simulink model "CM620C_MotAg0Meas"  (R2013b)
settings: Solver=FixedStepDiscrete  SolverMode=SingleTasking  StartTime=0.0  StopTime=1  FixedStep=0.0000625  RelTol=1e-3
values from neighbouring files (symbols this model uses):
  ARCHGLBPRM_2PI_ULS_F32 = DataDict.Constant    [CM620C_MotAg0Meas_DataDict.m]
  COEFFTBLELMSIZE_CNT_U08 = DataDict.Constant    [CM620C_MotAg0Meas_DataDict.m]
  COEFFTBLSIZE_CNT_U08 = DataDict.Constant    [CM620C_MotAg0Meas_DataDict.m]
  CORRNTBLAGSTEPSIZE_MATRAD_F32 = DataDict.Constant    [CM620C_MotAg0Meas_DataDict.m]
  CORRNTBLSIDXOFFS_CNT_U16 = DataDict.Constant    [CM620C_MotAg0Meas_DataDict.m]
  CORRNTBLSIZE_CNT_U16 = DataDict.Constant    [CM620C_MotAg0Meas_DataDict.m]
  CORRNTBLSIZEMASK_CNT_U08 = DataDict.Constant    [CM620C_MotAg0Meas_DataDict.m]
  MOTAG0ERRTHD_MOTREV_U0P16 = DataDict.Constant    [CM620C_MotAg0Meas_DataDict.m]
  MotAg0PrtclFlt = DataDict.NTC    [CM620C_MotAg0Meas_DataDict.m]
  MOTAG0PRTCLFLTFAILSTEP_CNT_U16 = DataDict.Constant    [CM620C_MotAg0Meas_DataDict.m]
  MOTAG0PRTCLFLTPASSSTEP_CNT_U16 = DataDict.Constant    [CM620C_MotAg0Meas_DataDict.m]
  MOTAGCPTLIMFLTMASK_CNT_U32 = DataDict.Constant    [CM620C_MotAg0Meas_DataDict.m]
  MOTAGDELTAPERCORRNPT_CNT_U16 = DataDict.Constant    [CM620C_MotAg0Meas_DataDict.m]
  MOTAGFLTMASK_CNT_U32 = DataDict.Constant    [CM620C_MotAg0Meas_DataDict.m]
  MOTAGIDXMASK_CNT_U16 = DataDict.Constant    [CM620C_MotAg0Meas_DataDict.m]
  MOTAGLIMMASK_CNT_S32 = DataDict.Constant    [CM620C_MotAg0Meas_DataDict.m]
  MOTAGMGNLIMFLTMASK_CNT_U32 = DataDict.Constant    [CM620C_MotAg0Meas_DataDict.m]
  MOTAGMINWAITPERD_CNT_U32 = DataDict.Constant    [CM620C_MotAg0Meas_DataDict.m]
  MOTAGOFFS_CNT_S32 = DataDict.Constant    [CM620C_MotAg0Meas_DataDict.m]
  MOTAGOVFFLTMASK_CNT_U32 = DataDict.Constant    [CM620C_MotAg0Meas_DataDict.m]
  MOTAGSPITRSMMASK_CNT_U32 = DataDict.Constant    [CM620C_MotAg0Meas_DataDict.m]
  MOTAGVLTGFLTMASK_CNT_U32 = DataDict.Constant    [CM620C_MotAg0Meas_DataDict.m]
  NOMOTAGFLTMASK_CNT_U32 = DataDict.Constant    [CM620C_MotAg0Meas_DataDict.m]
  READBUFADR_CNT_U32 = DataDict.Constant    [CM620C_MotAg0Meas_DataDict.m]
  READBUFIDX_CNT_U08 = DataDict.Constant    [CM620C_MotAg0Meas_DataDict.m]
  SNSRAGMASK_CNT_U32 = DataDict.Constant    [CM620C_MotAg0Meas_DataDict.m]
  SNSRCNTMASK_CNT_U32 = DataDict.Constant    [CM620C_MotAg0Meas_DataDict.m]
  SPIAGCNTREGIDX_CNT_U08 = DataDict.Constant    [CM620C_MotAg0Meas_DataDict.m]
  SPIAGREGIDX_CNT_U08 = DataDict.Constant    [CM620C_MotAg0Meas_DataDict.m]
  SPISTATREGIDX_CNT_U08 = DataDict.Constant    [CM620C_MotAg0Meas_DataDict.m]
  SPITURNCNTRREGIDX_CNT_U08 = DataDict.Constant    [CM620C_MotAg0Meas_DataDict.m]
  STRTPTRINITVAL_CNT_U32 = DataDict.Constant    [CM620C_MotAg0Meas_DataDict.m]
  STRTPTRPERVAL_CNT_U32 = DataDict.Constant    [CM620C_MotAg0Meas_DataDict.m]
  TURNCNTRHALFOFFS_CNT_S16 = DataDict.Constant    [CM620C_MotAg0Meas_DataDict.m]
  TURNCNTROFFS_CNT_S16 = DataDict.Constant    [CM620C_MotAg0Meas_DataDict.m]
  TURNCNTRREGMASK_CNT_U32 = DataDict.Constant    [CM620C_MotAg0Meas_DataDict.m]
  VLDMOTAGFLTMASK_CNT_U32 = DataDict.Constant    [CM620C_MotAg0Meas_DataDict.m]
undefined symbols (not defined in the file or in its folder): NtcSts1, sigbuilder_block
libraries: simulink x41, FloatToFixd x1, NxtrMax x1
(part 5 of 7)

== system CM620C_MotAg0Meas/MotAg0Meas/MotAg0MeasPer2/MotAg0Calcn/MotAg0Processing/Diagnostics/SetParamByte/Boolean to u8   ==
  InputBoolean : Inport  OutDataTypeStr=boolean
  CopyRight2 : Subsystem  Description=|  mask(Copyright Information){none=on}
      | Copyright info block.                                               
      |                                                                     
      | Place copyright information at the top of every subsystem in design.
      mask prompts: none "No parameters"
      mask help: Place copyright information at the top of every subsystem in design.
      mask Display:
      | NxtrConf = 'Nexteer Confidential';
      | 
      | sys = bdroot; %handle for the current model ("system")
      | first = get_param(sys,'Created');
      | first = first(end-3:end);  %year is last four digits
      | 
      | last = get_param(sys,'LastModifiedDate');
      | if isempty(last)
      |     last = datestr(now,'yyyy');
      | else
      |     last = last(end-3:end);
      | end
      | 
      | if strcmp(first,last)
      |     fprintf('%s -- Copyright %s Nexteer',NxtrConf,first)
      | else
      |     fprintf('%s -- %s%s- %s Nexteer',NxtrConf,char(169),first,last)
      | end
  If : If  IfExpression=u1 ~= 0
  Merge : Merge
  Output 0 : Subsystem  TreatAsAtomicUnit=on
  Output 1 : Subsystem  TreatAsAtomicUnit=on
  OutputNumber : Outport  OutDataTypeStr=uint8
  wires:
  InputBoolean/1 -> If/1
  If/1 -> Output 1/Action
  If/2 -> Output 0/Action
  Output 1/1(Out1) -> Merge/1
  Output 0/1(Out1) -> Merge/2
  Merge/1 -> OutputNumber/1

== system CM620C_MotAg0Meas/MotAg0Meas/MotAg0MeasPer2/MotAg0Calcn/MotAg0Processing/Diagnostics/SetParamByte/Boolean to u8    ==
  InputBoolean : Inport  OutDataTypeStr=boolean
  CopyRight2 : Subsystem  Description=|  mask(Copyright Information){none=on}
      | Copyright info block.                                               
      |                                                                     
      | Place copyright information at the top of every subsystem in design.
      mask prompts: none "No parameters"
      mask help: Place copyright information at the top of every subsystem in design.
      mask Display:
      | NxtrConf = 'Nexteer Confidential';
      | 
      | sys = bdroot; %handle for the current model ("system")
      | first = get_param(sys,'Created');
      | first = first(end-3:end);  %year is last four digits
      | 
      | last = get_param(sys,'LastModifiedDate');
      | if isempty(last)
      |     last = datestr(now,'yyyy');
      | else
      |     last = last(end-3:end);
      | end
      | 
      | if strcmp(first,last)
      |     fprintf('%s -- Copyright %s Nexteer',NxtrConf,first)
      | else
      |     fprintf('%s -- %s%s- %s Nexteer',NxtrConf,char(169),first,last)
      | end
  If : If  IfExpression=u1 ~= 0
  Merge : Merge
  Output 0 : Subsystem  TreatAsAtomicUnit=on
  Output 1 : Subsystem  TreatAsAtomicUnit=on
  OutputNumber : Outport  OutDataTypeStr=uint8
  wires:
  Merge/1 -> OutputNumber/1
  Output 0/1(Out1) -> Merge/2
  Output 1/1(Out1) -> Merge/1
  If/2 -> Output 0/Action
  If/1 -> Output 1/Action
  InputBoolean/1 -> If/1

== system CM620C_MotAg0Meas/MotAg0Meas/MotAg0MeasPer2/MotAg0Calcn/MotAg0Processing/Diagnostics/SetParamByte/Boolean to u8     ==
  InputBoolean : Inport  OutDataTypeStr=boolean
  CopyRight2 : Subsystem  Description=|  mask(Copyright Information){none=on}
      | Copyright info block.                                               
      |                                                                     
      | Place copyright information at the top of every subsystem in design.
      mask prompts: none "No parameters"
      mask help: Place copyright information at the top of every subsystem in design.
      mask Display:
      | NxtrConf = 'Nexteer Confidential';
      | 
      | sys = bdroot; %handle for the current model ("system")
      | first = get_param(sys,'Created');
      | first = first(end-3:end);  %year is last four digits
      | 
      | last = get_param(sys,'LastModifiedDate');
      | if isempty(last)
      |     last = datestr(now,'yyyy');
      | else
      |     last = last(end-3:end);
      | end
      | 
      | if strcmp(first,last)
      |     fprintf('%s -- Copyright %s Nexteer',NxtrConf,first)
      | else
      |     fprintf('%s -- %s%s- %s Nexteer',NxtrConf,char(169),first,last)
      | end
  If : If  IfExpression=u1 ~= 0
  Merge : Merge
  Output 0 : Subsystem  TreatAsAtomicUnit=on
  Output 1 : Subsystem  TreatAsAtomicUnit=on
  OutputNumber : Outport  OutDataTypeStr=uint8
  wires:
  InputBoolean/1 -> If/1
  If/1 -> Output 1/Action
  If/2 -> Output 0/Action
  Output 1/1(Out1) -> Merge/1
  Output 0/1(Out1) -> Merge/2
  Merge/1 -> OutputNumber/1

== system CM620C_MotAg0Meas/MotAg0Meas/MotAg0MeasPer2/MotAg0Calcn/MotAg0Processing/Diagnostics/SetParamByte/Boolean to u8      ==
  InputBoolean : Inport  OutDataTypeStr=boolean
  CopyRight2 : Subsystem  Description=|  mask(Copyright Information){none=on}
      | Copyright info block.                                               
      |                                                                     
      | Place copyright information at the top of every subsystem in design.
      mask prompts: none "No parameters"
      mask help: Place copyright information at the top of every subsystem in design.
      mask Display:
      | NxtrConf = 'Nexteer Confidential';
      | 
      | sys = bdroot; %handle for the current model ("system")
      | first = get_param(sys,'Created');
      | first = first(end-3:end);  %year is last four digits
      | 
      | last = get_param(sys,'LastModifiedDate');
      | if isempty(last)
      |     last = datestr(now,'yyyy');
      | else
      |     last = last(end-3:end);
      | end
      | 
      | if strcmp(first,last)
      |     fprintf('%s -- Copyright %s Nexteer',NxtrConf,first)
      | else
      |     fprintf('%s -- %s%s- %s Nexteer',NxtrConf,char(169),first,last)
      | end
  If : If  IfExpression=u1 ~= 0
  Merge : Merge
  Output 0 : Subsystem  TreatAsAtomicUnit=on
  Output 1 : Subsystem  TreatAsAtomicUnit=on
  OutputNumber : Outport  OutDataTypeStr=uint8
  wires:
  Merge/1 -> OutputNumber/1
  Output 0/1(Out1) -> Merge/2
  Output 1/1(Out1) -> Merge/1
  If/2 -> Output 0/Action
  If/1 -> Output 1/Action
  InputBoolean/1 -> If/1

== system CM620C_MotAg0Meas/MotAg0Meas/MotAg0MeasPer2/MotAg0Calcn/MotAg0Processing/Diagnostics/SetParamByte/Boolean to uint8 ==
  InputBoolean : Inport  OutDataTypeStr=boolean
  CopyRight2 : Subsystem  Description=|  mask(Copyright Information){none=on}
      | Copyright info block.                                               
      |                                                                     
      | Place copyright information at the top of every subsystem in design.
      mask prompts: none "No parameters"
      mask help: Place copyright information at the top of every subsystem in design.
      mask Display:
      | NxtrConf = 'Nexteer Confidential';
      | 
      | sys = bdroot; %handle for the current model ("system")
      | first = get_param(sys,'Created');
      | first = first(end-3:end);  %year is last four digits
      | 
      | last = get_param(sys,'LastModifiedDate');
      | if isempty(last)
      |     last = datestr(now,'yyyy');
      | else
      |     last = last(end-3:end);
      | end
      | 
      | if strcmp(first,last)
      |     fprintf('%s -- Copyright %s Nexteer',NxtrConf,first)
      | else
      |     fprintf('%s -- %s%s- %s Nexteer',NxtrConf,char(169),first,last)
      | end
  If : If  IfExpression=u1 ~= 0
  Merge : Merge
  Output 0 : Subsystem  TreatAsAtomicUnit=on
  Output 1 : Subsystem  TreatAsAtomicUnit=on
  OutputNumber : Outport  OutDataTypeStr=uint8
  wires:
  Merge/1 -> OutputNumber/1
  Output 0/1(Out1) -> Merge/2
  Output 1/1(Out1) -> Merge/1
  If/2 -> Output 0/Action
  If/1 -> Output 1/Action
  InputBoolean/1 -> If/1

== system CM620C_MotAg0Meas/MotAg0Meas/MotAg0MeasPer2/MotAg0Calcn/MotAg0Processing/Diagnostics/SetParamByte/CopyRight2 ==

== system CM620C_MotAg0Meas/MotAg0Meas/MotAg0MeasPer2/MotAg0Calcn/MotAg0Processing/Diagnostics/SetParamByte/Subsystem1 ==
  Test_Lgc : Inport
  MotAg0SyncErr : Inport  Port=2
  MotAg0NoAg : Inport  Port=3
  MotAg0NoXY : Inport  Port=4
  MotAg0OutofLim : Inport  Port=5
  MotAg0XYOutofLim : Inport  Port=6
  MotAg0DSPOverFlow : Inport  Port=7
  MotAg0VltgFlt : Inport  Port=8
  CopyRight2 : Subsystem  Description=|  mask(Copyright Information){none=on}
      | Copyright info block.                                               
      |                                                                     
      | Place copyright information at the top of every subsystem in design.
      mask prompts: none "No parameters"
      mask help: Place copyright information at the top of every subsystem in design.
      mask Display:
      | NxtrConf = 'Nexteer Confidential';
      | 
      | sys = bdroot; %handle for the current model ("system")
      | first = get_param(sys,'Created');
      | first = first(end-3:end);  %year is last four digits
      | 
      | last = get_param(sys,'LastModifiedDate');
      | if isempty(last)
      |     last = datestr(now,'yyyy');
      | else
      |     last = last(end-3:end);
      | end
      | 
      | if strcmp(first,last)
      |     fprintf('%s -- Copyright %s Nexteer',NxtrConf,first)
      | else
      |     fprintf('%s -- %s%s- %s Nexteer',NxtrConf,char(169),first,last)
      | end
  If : If  IfExpression=u1==1
  Merge : Merge
  No Fault : Subsystem  TreatAsAtomicUnit=on
  Scope : Scope
      settings: SaveName=ScopeData11
  Set ParamByte : Subsystem  TreatAsAtomicUnit=on
  ParamByte : Outport
  wires:
  MotAg0NoAg/1 -> Set ParamByte/1(MotAg0NoAg)
  MotAg0NoXY/1 -> Set ParamByte/2(MotAg0NoXY)
  MotAg0OutofLim/1 -> Set ParamByte/3(MotAg0OutofLim)
  MotAg0XYOutofLim/1 -> Set ParamByte/4(MotAg0XYOutofLim)
  MotAg0DSPOverFlow/1 -> Set ParamByte/5(MotAg0DSPOverFlow)
  MotAg0VltgFlt/1 -> Set ParamByte/6(MotAg0VltgFlt)
  Test_Lgc/1 -> If/1
  MotAg0SyncErr/1 -> Set ParamByte/7(MotAg0SyncErr)
  If/1 -> Set ParamByte/Action
  If/2 -> No Fault/Action
  Set ParamByte/1(ParamByte) -> Merge/1
  No Fault/1(ParamByte) -> Merge/2
  Merge/1 -> Scope/1, ParamByte/1

== system CM620C_MotAg0Meas/MotAg0Meas/MotAg0MeasPer2/MotAg0Calcn/MotAg0Processing/Offset Compensation /First Time Offset Calcn/CopyRight2 ==

== system CM620C_MotAg0Meas/MotAg0Meas/MotAg0MeasPer2/MotAg0Calcn/MotAg0Processing/Offset Compensation /Rt Offs Calcn/CopyRight2 ==

== system CM620C_MotAg0Meas/MotAg0Meas/MotAg0MeasPer2/MotAg0Calcn/MotAg0Processing/SPI  Motor Angle Calcn/Polarity Correction/CopyRight1 ==

== system CM620C_MotAg0Meas/MotAg0Meas/MotAg0MeasPer2/MotAg0Calcn/MotAg0Processing/SPI  Motor Angle Calcn/Polarity Correction/Negative Polarity ==
  MotAg0RawSpiMecl : Inport
  Action Port : ActionPort  ActionType=then
  Constant : Constant  Value=65535  OutDataTypeStr=uint16
  CopyRight2 : Subsystem  Description=|  mask(Copyright Information){none=on}
      | Copyright info block.                                               
      |                                                                     
      | Place copyright information at the top of every subsystem in design.
      mask prompts: none "No parameters"
      mask help: Place copyright information at the top of every subsystem in design.
      mask Display:
      | NxtrConf = 'Nexteer Confidential';
      | 
      | sys = bdroot; %handle for the current model ("system")
      | first = get_param(sys,'Created');
      | first = first(end-3:end);  %year is last four digits
      | 
      | last = get_param(sys,'LastModifiedDate');
      | if isempty(last)
      |     last = datestr(now,'yyyy');
      | else
      |     last = last(end-3:end);
      | end
      | 
      | if strcmp(first,last)
      |     fprintf('%s -- Copyright %s Nexteer',NxtrConf,first)
      | else
      |     fprintf('%s -- %s%s- %s Nexteer',NxtrConf,char(169),first,last)
      | end
  Subtract : Sum  Inputs=+-
  MotAg0SpiPolarityCorrd : Outport
  wires:
  Constant/1 -> Subtract/1
  MotAg0RawSpiMecl/1 -> Subtract/2
  Subtract/1 -> MotAg0SpiPolarityCorrd/1

== system CM620C_MotAg0Meas/MotAg0Meas/MotAg0MeasPer2/MotAg0Calcn/MotAg0Processing/SPI  Motor Angle Calcn/Polarity Correction/Positive Polarity ==
  MotAg0RawSpiMecl : Inport
  Action Port : ActionPort  ActionType=else
  CopyRight2 : Subsystem  Description=|  mask(Copyright Information){none=on}
      | Copyright info block.                                               
      |                                                                     
      | Place copyright information at the top of every subsystem in design.
      mask prompts: none "No parameters"
      mask help: Place copyright information at the top of every subsystem in design.
      mask Display:
      | NxtrConf = 'Nexteer Confidential';
      | 
      | sys = bdroot; %handle for the current model ("system")
      | first = get_param(sys,'Created');
      | first = first(end-3:end);  %year is last four digits
      | 
      | last = get_param(sys,'LastModifiedDate');
      | if isempty(last)
      |     last = datestr(now,'yyyy');
      | else
      |     last = last(end-3:end);
      | end
      | 
      | if strcmp(first,last)
      |     fprintf('%s -- Copyright %s Nexteer',NxtrConf,first)
      | else
      |     fprintf('%s -- %s%s- %s Nexteer',NxtrConf,char(169),first,last)
      | end
  MotAg0SpiPolarityCorrd : Outport
  wires:
  MotAg0RawSpiMecl/1 -> MotAg0SpiPolarityCorrd/1

== system CM620C_MotAg0Meas/MotAg0Meas/MotAg0MeasPer2/MotAg0Calcn/MotAg0Processing/SPI IIF Motor Angle/SpiMotAgCnt/CopyRight2 ==

== system CM620C_MotAg0Meas/MotAg0Meas/MotAg0MeasPer2/MotAg0Calcn/MotAg0Processing/Turns Counter Calcn/Negative Number/CopyRight2 ==

== system CM620C_MotAg0Meas/MotAg0Meas/MotAg0MeasPer2/MotAg0Calcn/MotAg0Processing/Turns Counter Calcn/Positive Number/CopyRight2 ==

== system CM620C_MotAg0Meas/MotAg0Meas/MotAg0MeasPer3/Initial Check/IdleState SendTx/Flt Cntr Ena/Wrap back to 0/CopyRight2 ==

== system CM620C_MotAg0Meas/MotAg0Meas/MotAg0MeasPer3/Initial Check/IdleState SendTx/Flt Cntr Ena/i++/CopyRight2 ==

== system CM620C_MotAg0Meas/MotAg0Meas/MotAg0MeasPer3/Initial Check/IdleState SendTx/MotAg0Sync/GetMotAg3Mecl/CopyRight2 ==

== system CM620C_MotAg0Meas/MotAg0Meas/MotAg0MeasPer3/Initial Check/IdleState SendTx/MotAg0Sync/IoHwAb_SetFctGpioMotAg0/CopyRight2 ==

== system CM620C_MotAg0Meas/MotAg0Meas/MotAg0MeasPer3/Initial Check/IdleState SendTx/MotAg0Sync/IoHwAb_SetFctPrphlMotAg0/CopyRight2 ==

== system CM620C_MotAg0Meas/MotAg0Meas/MotAg0MeasPer3/Initial Check/IdleState SendTx/MotAg0Sync/Set Chip Select High/CopyRight2 ==

== system CM620C_MotAg0Meas/MotAg0Meas/MotAg0MeasPer3/Initial Check/IdleState SendTx/MotAg0Sync/Set Chip Select High/IoHwAb_SetGpioMotAg0Cs ==
  PinSt : Inport  OutDataTypeStr=boolean
  CopyRight2 : Subsystem  Description=|  mask(Copyright Information){none=on}
      | Copyright info block.                                               
      |                                                                     
      | Place copyright information at the top of every subsystem in design.
      mask prompts: none "No parameters"
      mask help: Place copyright information at the top of every subsystem in design.
      mask Display:
      | NxtrConf = 'Nexteer Confidential';
      | 
      | sys = bdroot; %handle for the current model ("system")
      | first = get_param(sys,'Created');
      | first = first(end-3:end);  %year is last four digits
      | 
      | last = get_param(sys,'LastModifiedDate');
      | if isempty(last)
      |     last = datestr(now,'yyyy');
      | else
      |     last = last(end-3:end);
      | end
      | 
      | if strcmp(first,last)
      |     fprintf('%s -- Copyright %s Nexteer',NxtrConf,first)
      | else
      |     fprintf('%s -- %s%s- %s Nexteer',NxtrConf,char(169),first,last)
      | end
  Terminator : Terminator
  wires:
  PinSt/1 -> Terminator/1

== system CM620C_MotAg0Meas/MotAg0Meas/MotAg0MeasPer3/Initial Check/IdleState SendTx/MotAg0Sync/Set Chip Select Low/CopyRight2 ==

== system CM620C_MotAg0Meas/MotAg0Meas/MotAg0MeasPer3/Initial Check/IdleState SendTx/MotAg0Sync/Set Chip Select Low/IoHwAb_SetGpioMotAg0Cs ==
  PinSt : Inport  OutDataTypeStr=boolean
  CopyRight2 : Subsystem  Description=|  mask(Copyright Information){none=on}
      | Copyright info block.                                               
      |                                                                     
      | Place copyright information at the top of every subsystem in design.
      mask prompts: none "No parameters"
      mask help: Place copyright information at the top of every subsystem in design.
      mask Display:
      | NxtrConf = 'Nexteer Confidential';
      | 
      | sys = bdroot; %handle for the current model ("system")
      | first = get_param(sys,'Created');
      | first = first(end-3:end);  %year is last four digits
      | 
      | last = get_param(sys,'LastModifiedDate');
      | if isempty(last)
      |     last = datestr(now,'yyyy');
      | else
      |     last = last(end-3:end);
      | end
      | 
      | if strcmp(first,last)
      |     fprintf('%s -- Copyright %s Nexteer',NxtrConf,first)
      | else
      |     fprintf('%s -- %s%s- %s Nexteer',NxtrConf,char(169),first,last)
      | end
  Terminator : Terminator
  wires:
  PinSt/1 -> Terminator/1

== system CM620C_MotAg0Meas/MotAg0Meas/MotAg0MeasPer3/Initial Check/IdleState SendTx/MotAg0Sync/SpiTx/CopyRight2 ==

== system CM620C_MotAg0Meas/MotAg0Meas/MotAg0MeasPer3/Initial Check/IdleState SendTx/MotAg0Sync/Wait for 2us/CopyRight2 ==

== system CM620C_MotAg0Meas/MotAg0Meas/MotAg0MeasPer3/Initial Check/IdleState SendTx/MotAg0Sync/Wait for 2us/GetRefTmr1MicroSec32bit ==
  note: Dont code, simulation purposes only
  CopyRight2 : Subsystem  Description=|  mask(Copyright Information){none=on}
      | Copyright info block.                                               
      |                                                                     
      | Place copyright information at the top of every subsystem in design.
      mask prompts: none "No parameters"
      mask help: Place copyright information at the top of every subsystem in design.
      mask Display:
      | NxtrConf = 'Nexteer Confidential';
      | 
      | sys = bdroot; %handle for the current model ("system")
      | first = get_param(sys,'Created');
      | first = first(end-3:end);  %year is last four digits
      | 
      | last = get_param(sys,'LastModifiedDate');
      | if isempty(last)
      |     last = datestr(now,'yyyy');
      | else
      |     last = last(end-3:end);
      | end
      | 
      | if strcmp(first,last)
      |     fprintf('%s -- Copyright %s Nexteer',NxtrConf,first)
      | else
      |     fprintf('%s -- %s%s- %s Nexteer',NxtrConf,char(169),first,last)
      | end
  Data Type Conversion : DataTypeConversion  OutDataTypeStr=uint32
  Gain : Gain  Gain=1000000
  SystemTime : DigitalClock  RequirementInfo={} %GIDa_6e66b472_b7ad_4e9d_9794_91722c001009  SampleTime=-1
  RefTmr : Outport
  wires:
  SystemTime/1 -> Gain/1
  Gain/1 -> Data Type Conversion/1
  Data Type Conversion/1 -> RefTmr/1

== system CM620C_MotAg0Meas/MotAg0Meas/MotAg0MeasPer3/Initial Check/IdleState SendTx/MotAg0Sync/Wait for 2us/GetTiSpan1MicroSec32bit ==
  RefTmr : Inport
  CopyRight2 : Subsystem  Description=|  mask(Copyright Information){none=on}
      | Copyright info block.                                               
      |                                                                     
      | Place copyright information at the top of every subsystem in design.
      mask prompts: none "No parameters"
      mask help: Place copyright information at the top of every subsystem in design.
      mask Display:
      | NxtrConf = 'Nexteer Confidential';
      | 
      | sys = bdroot; %handle for the current model ("system")
      | first = get_param(sys,'Created');
      | first = first(end-3:end);  %year is last four digits
      | 
      | last = get_param(sys,'LastModifiedDate');
      | if isempty(last)
      |     last = datestr(now,'yyyy');
      | else
      |     last = last(end-3:end);
      | end
      | 
      | if strcmp(first,last)
      |     fprintf('%s -- Copyright %s Nexteer',NxtrConf,first)
      | else
      |     fprintf('%s -- %s%s- %s Nexteer',NxtrConf,char(169),first,last)
      | end
  Ground : Ground
  Terminator : Terminator
  TiSpan : Outport
  wires:
  RefTmr/1 -> Terminator/1
  Ground/1 -> TiSpan/1

== system CM620C_MotAg0Meas/MotAg0Meas/MotAg0MeasInit1/Compute Correction Table/NVM Ok/Calculate Correction Table/Build Wave/Reconstructed Waveform Processing/CopyRight2 ==

== system CM620C_MotAg0Meas/MotAg0Meas/MotAg0MeasInit1/Compute Correction Table/NVM Ok/Calculate Correction Table/Build Wave/Reconstructed Waveform Processing/Harmonic Coefficient Processing ==
  note: B coeff
  note: A coeff
  note: The Harmonic Coefficient Table
      | is constructed as 1D array with
      | the following format:
      |
      | tbl_00 = A0
      | tbl_01 = B0
      | tbl_02 = A1
      | tbl_03 = B1
      | tbl_04 = A2
      | tbl_05 = B2
      | tbl_06 = A3
      | tbl_07 = B3
      | ...
  HarmAngle : Inport
  Coefficient Table Size : Inport  Port=2
  Add : Sum  Inputs=+++
  Bias : Bias  Bias=+1
  Constant : Constant  Value=COEFFTBLELMSIZE_CNT_U08
  CopyRight2 : Subsystem  Description=|  mask(Copyright Information){none=on}
      | Copyright info block.                                               
      |                                                                     
      | Place copyright information at the top of every subsystem in design.
      mask prompts: none "No parameters"
      mask help: Place copyright information at the top of every subsystem in design.
      mask Display:
      | NxtrConf = 'Nexteer Confidential';
      | 
      | sys = bdroot; %handle for the current model ("system")
      | first = get_param(sys,'Created');
      | first = first(end-3:end);  %year is last four digits
      | 
      | last = get_param(sys,'LastModifiedDate');
      | if isempty(last)
      |     last = datestr(now,'yyyy');
      | else
      |     last = last(end-3:end);
      | end
      | 
      | if strcmp(first,last)
      |     fprintf('%s -- Copyright %s Nexteer',NxtrConf,first)
      | else
      |     fprintf('%s -- %s%s- %s Nexteer',NxtrConf,char(169),first,last)
      | end
  Data Store Read : DataStoreRead  DataStoreName=MotAg0CoeffTbl
  Data Type Conversion : DataTypeConversion  OutDataTypeStr=single
  Direct Lookup Table (n-D) : LookupNDDirect  NumberOfTableDimensions=1  TableIsInput=on
  Direct Lookup Table (n-D)1 : LookupNDDirect  NumberOfTableDimensions=1  TableIsInput=on
  For Iterator : ForIterator  ResetStates=reset  IterationSource=external  IterationVariableDataType=int8
  Product{,1..3} (4 alike) : Product
  SinCos (Use library function from NxtrMath) : Subsystem  TreatAsAtomicUnit=on
  Unit Delay : UnitDelay  SampleTime=-1
  Reconstructed Waveform Element : Outport
  wires:
  Coefficient Table Size/1 -> For Iterator/1
  Data Store Read/1 -> Direct Lookup Table (n-D)/2, Direct Lookup Table (n-D)1/2
  Constant/1 -> Product/2
  For Iterator/1 -> Data Type Conversion/1, Product/1
  HarmAngle/1 -> Product1/1
  Data Type Conversion/1 -> Product1/2
  Product1/1 -> SinCos (Use library function from NxtrMath)/1(Theta)
  Product/1 -> Bias/1, Direct Lookup Table (n-D)/1
  Bias/1 -> Direct Lookup Table (n-D)1/1
  SinCos (Use library function from NxtrMath)/2(Cos) -> Product2/1
  Direct Lookup Table (n-D)/1 -> Product2/2
  Direct Lookup Table (n-D)1/1 -> Product3/2
  SinCos (Use library function from NxtrMath)/1(Sin) -> Product3/1
  Product2/1 -> Add/1
  Product3/1 -> Add/2
  Unit Delay/1 -> Add/3
  Add/1 -> Unit Delay/1, Reconstructed Waveform Element/1

== system CM620C_MotAg0Meas/MotAg0Meas/MotAg0MeasInit1/Compute Correction Table/NVM Ok/Calculate Correction Table/Change Correction Coordinate/Waveform Coordinate Change/Calculate Index Scale ==
  Reconstructed Waveform_In : Inport
  LoopIndex : Inport  Port=2
  CopyRight2 : Subsystem  Description=|  mask(Copyright Information){none=on}
      | Copyright info block.                                               
      |                                                                     
      | Place copyright information at the top of every subsystem in design.
      mask prompts: none "No parameters"
      mask help: Place copyright information at the top of every subsystem in design.
      mask Display:
      | NxtrConf = 'Nexteer Confidential';
      | 
      | sys = bdroot; %handle for the current model ("system")
      | first = get_param(sys,'Created');
      | first = first(end-3:end);  %year is last four digits
      | 
      | last = get_param(sys,'LastModifiedDate');
      | if isempty(last)
      |     last = datestr(now,'yyyy');
      | else
      |     last = last(end-3:end);
      | end
      | 
      | if strcmp(first,last)
      |     fprintf('%s -- Copyright %s Nexteer',NxtrConf,first)
      | else
      |     fprintf('%s -- %s%s- %s Nexteer',NxtrConf,char(169),first,last)
      | end
  Direct Lookup Table (n-D) : LookupNDDirect  NumberOfTableDimensions=1  TableIsInput=on
  First Entry Index : Constant  Value=0
  First Entry Index1 : Constant  Value=ARCHGLBPRM_2PI_ULS_F32
  Truth Table : Truth Table  TreatAsAtomicUnit=on
  IndexScale : Outport
  wires:
  Reconstructed Waveform_In/1 -> Direct Lookup Table (n-D)/2
  First Entry Index/1 -> Direct Lookup Table (n-D)/1
  Direct Lookup Table (n-D)/1 -> Truth Table/1(ReconWfrm_0)
  LoopIndex/1 -> Truth Table/2(LoopIndex)
  First Entry Index1/1 -> Truth Table/3(ARCHGLBPRM_2PI_ULS_F32)
  Truth Table/1(IndexScale) -> IndexScale/1

== system CM620C_MotAg0Meas/MotAg0Meas/MotAg0MeasInit1/Compute Correction Table/NVM Ok/Calculate Correction Table/Change Correction Coordinate/Waveform Coordinate Change/CopyRight2 ==

== system CM620C_MotAg0Meas/MotAg0Meas/MotAg0MeasInit1/Compute Correction Table/NVM Ok/Calculate Correction Table/Change Correction Coordinate/Waveform Coordinate Change/Correction Term Found ==
  CorrnTerm_FoundIn : Inport
  Action Port : ActionPort  ActionType=else
  CopyRight2 : Subsystem  Description=|  mask(Copyright Information){none=on}
      | Copyright info block.                                               
      |                                                                     
      | Place copyright information at the top of every subsystem in design.
      mask prompts: none "No parameters"
      mask help: Place copyright information at the top of every subsystem in design.
      mask Display:
      | NxtrConf = 'Nexteer Confidential';
      | 
      | sys = bdroot; %handle for the current model ("system")
      | first = get_param(sys,'Created');
      | first = first(end-3:end);  %year is last four digits
      | 
      | last = get_param(sys,'LastModifiedDate');
      | if isempty(last)
      |     last = datestr(now,'yyyy');
      | else
      |     last = last(end-3:end);
      | end
      | 
      | if strcmp(first,last)
      |     fprintf('%s -- Copyright %s Nexteer',NxtrConf,first)
      | else
      |     fprintf('%s -- %s%s- %s Nexteer',NxtrConf,char(169),first,last)
      | end
  CorrnTerm_Found : Outport
  wires:
  CorrnTerm_FoundIn/1 -> CorrnTerm_Found/1

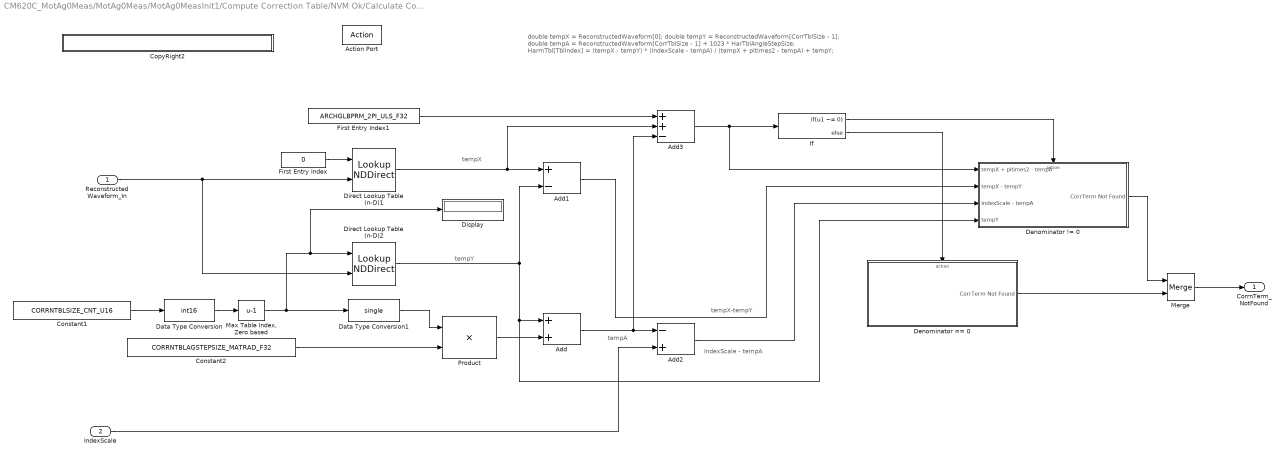
== system CM620C_MotAg0Meas/MotAg0Meas/MotAg0MeasInit1/Compute Correction Table/NVM Ok/Calculate Correction Table/Change Correction Coordinate/Waveform Coordinate Change/Correction Term Not Found ==
  note: double tempX = ReconstructedWaveform[0];
      | double tempY = ReconstructedWaveform[CorrTblSize - 1];
      | double tempA = ReconstructedWaveform[CorrTblSize - 1] + 1023 * HarTblAngleStepSize;
      |
      | HarmTbl[TblIndex] = (tempX - tempY) * (IndexScale - tempA) / (tempX + pitimes2 - tempA) + tempY;
  note: tempX-tempY
  note: IndexScale - tempA
  note: tempA
  note: tempX
  note: tempY
  Reconstructed Waveform_In : Inport  OutDataTypeStr=single
  IndexScale : Inport  Port=2
  Action Port : ActionPort  ActionType=then
  Add : Sum
  Add1 : Sum  Inputs=+-
  Add2 : Sum  Inputs=-+
  Add3 : Sum  Inputs=++-
  Constant1 : Constant  Value=CORRNTBLSIZE_CNT_U16
  Constant2 : Constant  Value=CORRNTBLAGSTEPSIZE_MATRAD_F32
  CopyRight2 : Subsystem  Description=|  mask(Copyright Information){none=on}
      | Copyright info block.                                               
      |                                                                     
      | Place copyright information at the top of every subsystem in design.
      mask prompts: none "No parameters"
      mask help: Place copyright information at the top of every subsystem in design.
      mask Display:
      | NxtrConf = 'Nexteer Confidential';
      | 
      | sys = bdroot; %handle for the current model ("system")
      | first = get_param(sys,'Created');
      | first = first(end-3:end);  %year is last four digits
      | 
      | last = get_param(sys,'LastModifiedDate');
      | if isempty(last)
      |     last = datestr(now,'yyyy');
      | else
      |     last = last(end-3:end);
      | end
      | 
      | if strcmp(first,last)
      |     fprintf('%s -- Copyright %s Nexteer',NxtrConf,first)
      | else
      |     fprintf('%s -- %s%s- %s Nexteer',NxtrConf,char(169),first,last)
      | end
  Data Type Conversion : DataTypeConversion  OutDataTypeStr=int16
  Data Type Conversion1 : DataTypeConversion  OutDataTypeStr=single
  Denominator != 0 : Subsystem  TreatAsAtomicUnit=on
  Denominator == 0 : Subsystem  TreatAsAtomicUnit=on
  Direct Lookup Table (n-D)1 : LookupNDDirect  NumberOfTableDimensions=1  TableIsInput=on
  Direct Lookup Table (n-D)2 : LookupNDDirect  NumberOfTableDimensions=1  TableIsInput=on
  Display : Display
  First Entry Index : Constant  Value=0
  First Entry Index1 : Constant  Value=ARCHGLBPRM_2PI_ULS_F32
  If : If  IfExpression=u1 ~= 0
  "Max Table Index, Zero based" : Bias  Bias=-1
  Merge : Merge
  Product : Product
  CorrnTerm_NotFound : Outport
  wires:
  Reconstructed Waveform_In/1 -> Direct Lookup Table (n-D)2/2, Direct Lookup Table (n-D)1/2
  First Entry Index/1 -> Direct Lookup Table (n-D)1/1
  Constant2/1 -> Product/2
  Constant1/1 -> Data Type Conversion/1
  "Max Table Index, Zero based"/1 -> Data Type Conversion1/1, Display/1, Direct Lookup Table (n-D)2/1
  Data Type Conversion/1 -> "Max Table Index, Zero based"/1
  Data Type Conversion1/1 -> Product/1
  Direct Lookup Table (n-D)2/1 -> Add1/2, Denominator != 0/4(tempY), Add/1
  Product/1 -> Add/2
  Direct Lookup Table (n-D)1/1 -> Add3/2, Add1/1
  Add/1 -> Add3/3, Add2/1
  IndexScale/1 -> Add2/2
  Add2/1 -> Denominator != 0/3(IndexScale - tempA)
  Add1/1 -> Denominator != 0/2(tempX - tempY)
  First Entry Index1/1 -> Add3/1
  If/1 -> Denominator != 0/Action
  If/2 -> Denominator == 0/Action
  Denominator != 0/1(CorrTerm Not Found) -> Merge/1
  Denominator == 0/1(CorrTerm Not Found) -> Merge/2
  Merge/1 -> CorrnTerm_NotFound/1
  Add3/1 -> Denominator != 0/1(tempX + pitimes2 - tempA), If/1

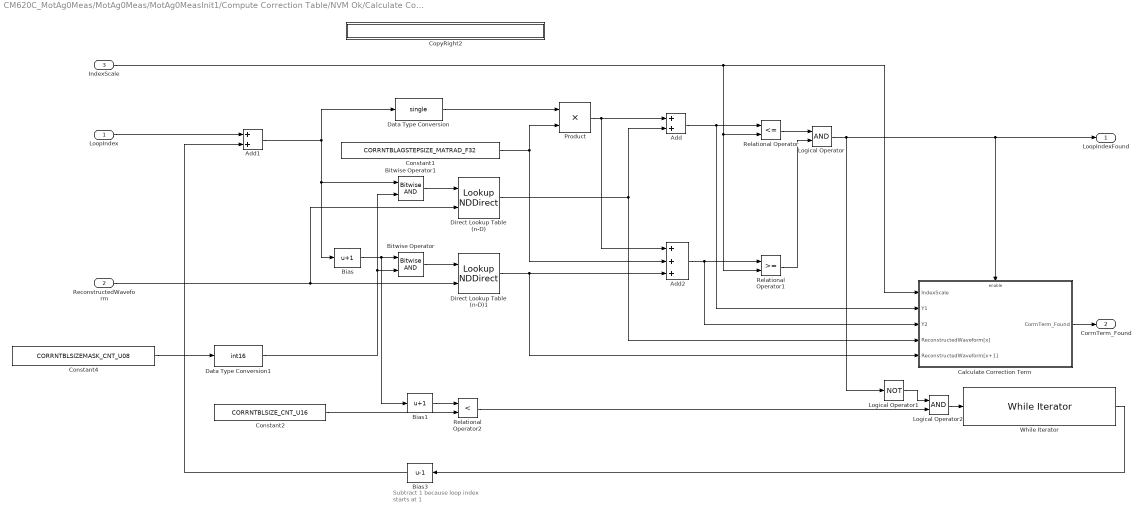
== system CM620C_MotAg0Meas/MotAg0Meas/MotAg0MeasInit1/Compute Correction Table/NVM Ok/Calculate Correction Table/Change Correction Coordinate/Waveform Coordinate Change/Determine Non Wrapped Correction Term ==
  note: Subtract 1 because
      | loop index starts at 1
  LoopIndex : Inport
  ReconstructedWaveform : Inport  Port=2
  IndexScale : Inport  Port=3
  Add : Sum
  Add1 : Sum
  Add2 : Sum  Inputs=+++
  Bias : Bias  Bias=1
  Bias1 : Bias  Bias=1
  Bias3 : Bias  Bias=-1
  Bitwise Operator : simulink/Logic and Bit Operations/Bitwise Operator  logicop=AND  UseBitMask=off  NumInputPorts=2  BitMask=CORRNTBLSIZE_CNT_U16-1  BitMaskRealWorld=Stored Integer
  Bitwise Operator1 : simulink/Logic and Bit Operations/Bitwise Operator  logicop=AND  UseBitMask=off  NumInputPorts=2  BitMask=CORRNTBLSIZE_CNT_U16-1  BitMaskRealWorld=Stored Integer
  Calculate Correction Term : Subsystem  TreatAsAtomicUnit=on
  Constant1 : Constant  Value=CORRNTBLAGSTEPSIZE_MATRAD_F32
  Constant2 : Constant  Value=CORRNTBLSIZE_CNT_U16
  Constant4 : Constant  Value=CORRNTBLSIZEMASK_CNT_U08
  CopyRight2 : Subsystem  Description=|  mask(Copyright Information){none=on}
      | Copyright info block.                                               
      |                                                                     
      | Place copyright information at the top of every subsystem in design.
      mask prompts: none "No parameters"
      mask help: Place copyright information at the top of every subsystem in design.
      mask Display:
      | NxtrConf = 'Nexteer Confidential';
      | 
      | sys = bdroot; %handle for the current model ("system")
      | first = get_param(sys,'Created');
      | first = first(end-3:end);  %year is last four digits
      | 
      | last = get_param(sys,'LastModifiedDate');
      | if isempty(last)
      |     last = datestr(now,'yyyy');
      | else
      |     last = last(end-3:end);
      | end
      | 
      | if strcmp(first,last)
      |     fprintf('%s -- Copyright %s Nexteer',NxtrConf,first)
      | else
      |     fprintf('%s -- %s%s- %s Nexteer',NxtrConf,char(169),first,last)
      | end
  Data Type Conversion : DataTypeConversion  OutDataTypeStr=single
  Data Type Conversion1 : DataTypeConversion  OutDataTypeStr=int16
  Direct Lookup Table (n-D) : LookupNDDirect  NumberOfTableDimensions=1  TableIsInput=on
  Direct Lookup Table (n-D)1 : LookupNDDirect  NumberOfTableDimensions=1  TableIsInput=on
  Logical Operator : Logic  AllPortsSameDT=off  OutDataTypeStr=boolean
  Logical Operator1 : Logic  Operator=NOT  AllPortsSameDT=off  OutDataTypeStr=boolean
  Logical Operator2 : Logic  AllPortsSameDT=off  OutDataTypeStr=boolean
  Product : Product
  Relational Operator : RelationalOperator  Operator=<=  OutDataTypeStr=boolean
  Relational Operator1 : RelationalOperator  OutDataTypeStr=boolean
  Relational Operator2 : RelationalOperator  Operator=<  OutDataTypeStr=boolean
  While Iterator : WhileIterator  MaxIters=128  WhileBlockType=do-while  ShowIterationPort=on  OutputDataType=int16
      settings: AttributesFormatString=|
      | Max Iterations:
      | %<MaxIters>
      | (CORRNTBLSIZE_CNT_U16)
  LoopIndexFound : Outport
  CorrnTerm_Found : Outport  Port=2
  wires:
  ReconstructedWaveform/1 -> Direct Lookup Table (n-D)/2, Direct Lookup Table (n-D)1/2
  Add1/1 -> Data Type Conversion/1, Bias/1, Bitwise Operator1/1
  Bias/1 -> Bias1/1, Bitwise Operator/1
  Data Type Conversion/1 -> Product/1
  Product/1 -> Add2/1, Add/1
  Direct Lookup Table (n-D)/1 -> Add/2, Calculate Correction Term/4(ReconstructedWaveform[x])
  LoopIndex/1 -> Add1/1
  Constant1/1 -> Product/2, Add2/2
  Direct Lookup Table (n-D)1/1 -> Calculate Correction Term/5(ReconstructedWaveform[x+1]), Add2/3
  Add/1 -> Calculate Correction Term/2(Y1), Relational Operator/1
  IndexScale/1 -> Calculate Correction Term/1(IndexScale), Relational Operator1/2, Relational Operator/2
  Add2/1 -> Calculate Correction Term/3(Y2), Relational Operator1/1
  Relational Operator/1 -> Logical Operator/1
  Relational Operator1/1 -> Logical Operator/2
  Logical Operator/1 -> Calculate Correction Term/Enable, LoopIndexFound/1, Logical Operator1/1
  Bitwise Operator/1 -> Direct Lookup Table (n-D)1/1
  Bitwise Operator1/1 -> Direct Lookup Table (n-D)/1
  Logical Operator1/1 -> Logical Operator2/1
  Relational Operator2/1 -> Logical Operator2/2
  Logical Operator2/1 -> While Iterator/1
  Constant2/1 -> Relational Operator2/2
  Bias1/1 -> Relational Operator2/1
  While Iterator/1 -> Bias3/1
  Bias3/1 -> Add1/2
  Calculate Correction Term/1(CorrnTerm_Found) -> CorrnTerm_Found/1
  Constant4/1 -> Data Type Conversion1/1
  Data Type Conversion1/1 -> Bitwise Operator/2, Bitwise Operator1/2

== system CM620C_MotAg0Meas/MotAg0Meas/MotAg0MeasPer2/MotAg0Calcn/MotAg0Processing/Diagnostics/ Qualifier Sts/GetNtcQlfr/CopyRight2 ==

== system CM620C_MotAg0Meas/MotAg0Meas/MotAg0MeasPer2/MotAg0Calcn/MotAg0Processing/Diagnostics/ Qualifier Sts/NtcSts and DebStep Calcn/CopyRight2 ==

== system CM620C_MotAg0Meas/MotAg0Meas/MotAg0MeasPer2/MotAg0Calcn/MotAg0Processing/Diagnostics/ Qualifier Sts/NtcSts and DebStep Calcn/N Step ==
  Action Port : ActionPort  ActionType=else
  CopyRight2 : Subsystem  Description=|  mask(Copyright Information){none=on}
      | Copyright info block.                                               
      |                                                                     
      | Place copyright information at the top of every subsystem in design.
      mask prompts: none "No parameters"
      mask help: Place copyright information at the top of every subsystem in design.
      mask Display:
      | NxtrConf = 'Nexteer Confidential';
      | 
      | sys = bdroot; %handle for the current model ("system")
      | first = get_param(sys,'Created');
      | first = first(end-3:end);  %year is last four digits
      | 
      | last = get_param(sys,'LastModifiedDate');
      | if isempty(last)
      |     last = datestr(now,'yyyy');
      | else
      |     last = last(end-3:end);
      | end
      | 
      | if strcmp(first,last)
      |     fprintf('%s -- Copyright %s Nexteer',NxtrConf,first)
      | else
      |     fprintf('%s -- %s%s- %s Nexteer',NxtrConf,char(169),first,last)
      | end
  NtcNr1 : simulink/Sources/Enumerated Constant  OutDataTypeStr=Enum: NtcSts1  Value=NtcSts1.NTCSTS_PREPASSD  SampleTime=inf
  PassStep 32767/50 : Constant  Value=MOTAG0PRTCLFLTPASSSTEP_CNT_U16  OutDataTypeStr=uint16
  NtcSts : Outport
  DebStep : Outport  Port=2
  wires:
  PassStep 32767/50/1 -> DebStep/1
  NtcNr1/1 -> NtcSts/1

== system CM620C_MotAg0Meas/MotAg0Meas/MotAg0MeasPer2/MotAg0Calcn/MotAg0Processing/Diagnostics/ Qualifier Sts/NtcSts and DebStep Calcn/P Step ==
  Action Port : ActionPort  ActionType=then
  CopyRight2 : Subsystem  Description=|  mask(Copyright Information){none=on}
      | Copyright info block.                                               
      |                                                                     
      | Place copyright information at the top of every subsystem in design.
      mask prompts: none "No parameters"
      mask help: Place copyright information at the top of every subsystem in design.
      mask Display:
      | NxtrConf = 'Nexteer Confidential';
      | 
      | sys = bdroot; %handle for the current model ("system")
      | first = get_param(sys,'Created');
      | first = first(end-3:end);  %year is last four digits
      | 
      | last = get_param(sys,'LastModifiedDate');
      | if isempty(last)
      |     last = datestr(now,'yyyy');
      | else
      |     last = last(end-3:end);
      | end
      | 
      | if strcmp(first,last)
      |     fprintf('%s -- Copyright %s Nexteer',NxtrConf,first)
      | else
      |     fprintf('%s -- %s%s- %s Nexteer',NxtrConf,char(169),first,last)
      | end
  "Fail Step 32767/10 " : Constant  Value=MOTAG0PRTCLFLTFAILSTEP_CNT_U16  OutDataTypeStr=uint16
  NtcNr1 : simulink/Sources/Enumerated Constant  OutDataTypeStr=Enum: NtcSts1  Value=NtcSts1.NTCSTS_PREFAILD  SampleTime=inf
  NtcSts : Outport
  DebStep : Outport  Port=2
  wires:
  NtcNr1/1 -> NtcSts/1
  "Fail Step 32767/10 "/1 -> DebStep/1

== system CM620C_MotAg0Meas/MotAg0Meas/MotAg0MeasPer2/MotAg0Calcn/MotAg0Processing/Diagnostics/ Qualifier Sts/SetNtcSts/CopyRight2 ==

== system CM620C_MotAg0Meas/MotAg0Meas/MotAg0MeasPer2/MotAg0Calcn/MotAg0Processing/Diagnostics/Rolling Counter/Test Faild/CopyRight2 ==

== system CM620C_MotAg0Meas/MotAg0Meas/MotAg0MeasPer2/MotAg0Calcn/MotAg0Processing/Diagnostics/Rolling Counter/Test Pass/CopyRight2 ==

== system CM620C_MotAg0Meas/MotAg0Meas/MotAg0MeasPer2/MotAg0Calcn/MotAg0Processing/Diagnostics/Rolling Counter/Test Pass/Wrap back to 0 ==
  Action Port : ActionPort  ActionType=then
  Constant : Constant  Value=0  OutDataTypeStr=uint8
  CopyRight2 : Subsystem  Description=|  mask(Copyright Information){none=on}
      | Copyright info block.                                               
      |                                                                     
      | Place copyright information at the top of every subsystem in design.
      mask prompts: none "No parameters"
      mask help: Place copyright information at the top of every subsystem in design.
      mask Display:
      | NxtrConf = 'Nexteer Confidential';
      | 
      | sys = bdroot; %handle for the current model ("system")
      | first = get_param(sys,'Created');
      | first = first(end-3:end);  %year is last four digits
      | 
      | last = get_param(sys,'LastModifiedDate');
      | if isempty(last)
      |     last = datestr(now,'yyyy');
      | else
      |     last = last(end-3:end);
      | end
      | 
      | if strcmp(first,last)
      |     fprintf('%s -- Copyright %s Nexteer',NxtrConf,first)
      | else
      |     fprintf('%s -- %s%s- %s Nexteer',NxtrConf,char(169),first,last)
      | end
  RollgCntr : Outport
  wires:
  Constant/1 -> RollgCntr/1

== system CM620C_MotAg0Meas/MotAg0Meas/MotAg0MeasPer2/MotAg0Calcn/MotAg0Processing/Diagnostics/Rolling Counter/Test Pass/i++ ==
  Action Port : ActionPort  ActionType=else
  Add : Sum
  Constant : Constant  OutDataTypeStr=uint8
  CopyRight2 : Subsystem  Description=|  mask(Copyright Information){none=on}
      | Copyright info block.                                               
      |                                                                     
      | Place copyright information at the top of every subsystem in design.
      mask prompts: none "No parameters"
      mask help: Place copyright information at the top of every subsystem in design.
      mask Display:
      | NxtrConf = 'Nexteer Confidential';
      | 
      | sys = bdroot; %handle for the current model ("system")
      | first = get_param(sys,'Created');
      | first = first(end-3:end);  %year is last four digits
      | 
      | last = get_param(sys,'LastModifiedDate');
      | if isempty(last)
      |     last = datestr(now,'yyyy');
      | else
      |     last = last(end-3:end);
      | end
      | 
      | if strcmp(first,last)
      |     fprintf('%s -- Copyright %s Nexteer',NxtrConf,first)
      | else
      |     fprintf('%s -- %s%s- %s Nexteer',NxtrConf,char(169),first,last)
      | end
  Data Store Read : DataStoreRead  DataStoreName=MotAg0PrevRollgCntr
  RollgCntr : Outport
  wires:
  Constant/1 -> Add/1
  Data Store Read/1 -> Add/2
  Add/1 -> RollgCntr/1

== system CM620C_MotAg0Meas/MotAg0Meas/MotAg0MeasPer2/MotAg0Calcn/MotAg0Processing/Diagnostics/SPI vs ENCA/No Error/CopyRight2 ==

== system CM620C_MotAg0Meas/MotAg0Meas/MotAg0MeasPer2/MotAg0Calcn/MotAg0Processing/Diagnostics/SPI vs ENCA/Sub 0/CopyRight2 ==

== system CM620C_MotAg0Meas/MotAg0Meas/MotAg0MeasPer2/MotAg0Calcn/MotAg0Processing/Diagnostics/SPI vs ENCA/Sub 65535/CopyRight2 ==

== system CM620C_MotAg0Meas/MotAg0Meas/MotAg0MeasPer2/MotAg0Calcn/MotAg0Processing/Diagnostics/SPI vs ENCA/Sync Error/CopyRight2 ==

== system CM620C_MotAg0Meas/MotAg0Meas/MotAg0MeasPer2/MotAg0Calcn/MotAg0Processing/Diagnostics/SetParamByte/Boolean to u8/CopyRight2 ==

== system CM620C_MotAg0Meas/MotAg0Meas/MotAg0MeasPer2/MotAg0Calcn/MotAg0Processing/Diagnostics/SetParamByte/Boolean to u8/Output 0 ==
  Action Port : ActionPort  ActionType=else
  Bit 7 : Constant  Value=0  OutDataTypeStr=uint8
  CopyRight2 : Subsystem  Description=|  mask(Copyright Information){none=on}
      | Copyright info block.                                               
      |                                                                     
      | Place copyright information at the top of every subsystem in design.
      mask prompts: none "No parameters"
      mask help: Place copyright information at the top of every subsystem in design.
      mask Display:
      | NxtrConf = 'Nexteer Confidential';
      | 
      | sys = bdroot; %handle for the current model ("system")
      | first = get_param(sys,'Created');
      | first = first(end-3:end);  %year is last four digits
      | 
      | last = get_param(sys,'LastModifiedDate');
      | if isempty(last)
      |     last = datestr(now,'yyyy');
      | else
      |     last = last(end-3:end);
      | end
      | 
      | if strcmp(first,last)
      |     fprintf('%s -- Copyright %s Nexteer',NxtrConf,first)
      | else
      |     fprintf('%s -- %s%s- %s Nexteer',NxtrConf,char(169),first,last)
      | end
  Out1 : Outport  InitialOutput=0
  wires:
  Bit 7/1 -> Out1/1

== system CM620C_MotAg0Meas/MotAg0Meas/MotAg0MeasPer2/MotAg0Calcn/MotAg0Processing/Diagnostics/SetParamByte/Boolean to u8/Output 1 ==
  Action Port : ActionPort  ActionType=then
  Bit 7 : Constant  OutDataTypeStr=uint8
  CopyRight2 : Subsystem  Description=|  mask(Copyright Information){none=on}
      | Copyright info block.                                               
      |                                                                     
      | Place copyright information at the top of every subsystem in design.
      mask prompts: none "No parameters"
      mask help: Place copyright information at the top of every subsystem in design.
      mask Display:
      | NxtrConf = 'Nexteer Confidential';
      | 
      | sys = bdroot; %handle for the current model ("system")
      | first = get_param(sys,'Created');
      | first = first(end-3:end);  %year is last four digits
      | 
      | last = get_param(sys,'LastModifiedDate');
      | if isempty(last)
      |     last = datestr(now,'yyyy');
      | else
      |     last = last(end-3:end);
      | end
      | 
      | if strcmp(first,last)
      |     fprintf('%s -- Copyright %s Nexteer',NxtrConf,first)
      | else
      |     fprintf('%s -- %s%s- %s Nexteer',NxtrConf,char(169),first,last)
      | end
  Out1 : Outport  InitialOutput=1
  wires:
  Bit 7/1 -> Out1/1

== system CM620C_MotAg0Meas/MotAg0Meas/MotAg0MeasPer2/MotAg0Calcn/MotAg0Processing/Diagnostics/SetParamByte/Boolean to u8 /CopyRight2 ==
